simulink library "ILCUpdate"  (R2018a)
settings: Solver=VariableStepAuto  StartTime=0.0  StopTime=10.0  RelTol=1e-3
undefined symbols (not defined in the file or in its folder): ctrl
libraries: normalizeBasisParameters x2, updateLaw_cd x1, initializeResponseSurface_cd x1, manageILCTriggers_ul x1, updateResponseSurface_ul x1, normalizePerformanceIndex x1, rescaleBasisParameters x1
settings Model: Creator=mitch  LastModifiedBy=mitch

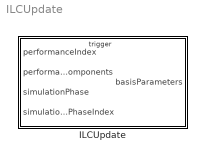
== system ILCUpdate ==
  ILCUpdate : Subsystem

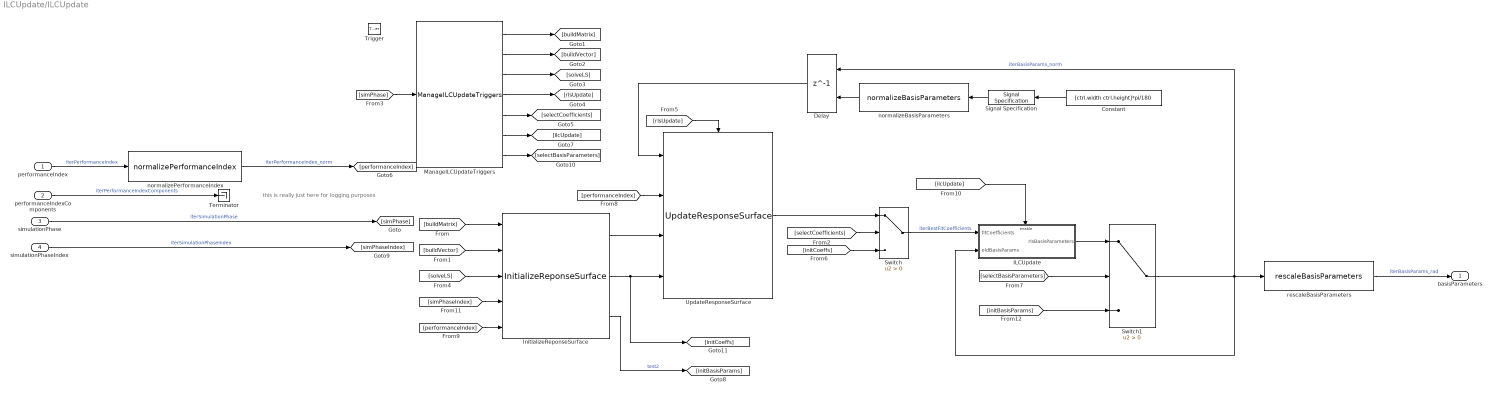
== system ILCUpdate/ILCUpdate ==
  note: this is really just here for logging purposes
  performanceIndex : Inport
  performanceIndexComponents : Inport  Port=2
  simulationPhase : Inport  Port=3  OutDataTypeStr=Enum: simulationPhase_enum
  simulationPhaseIndex : Inport  Port=4
  Trigger : TriggerPort  VariantControl=Variant  InitialTriggerSignalState=positive  PortDimensions=1
  Constant : Constant  Value=[ctrl.width ctrl.height]*pi/180
  Delay : Delay  DelayLength=1  InitialConditionSource=Input port
      settings: InputPortMap=u0,p4
  ILCUpdate : Subsystem
  InitializeReponseSurface : initializeResponseSurface_cd/InitializeReponseSurface
  ManageILCUpdateTriggers : manageILCTriggers_ul/ManageILCUpdateTriggers
  Signal Specification : SignalSpecification  Dimensions=[1 2]
  Switch : Switch  Criteria=u2 > Threshold
  Switch1 : Switch  Criteria=u2 > Threshold
  Terminator : Terminator
  UpdateResponseSurface : updateResponseSurface_ul/UpdateResponseSurface
  normalizeBasisParameters : normalizeBasisParameters/normalizeBasisParameters
  normalizePerformanceIndex : normalizePerformanceIndex/normalizePerformanceIndex
  rescaleBasisParameters : rescaleBasisParameters/rescaleBasisParameters
  basisParameters : Outport  InitialOutput=[ctrl.width ctrl.height]*pi/180
  wires:
  [initBasisParams] -> Switch1/3
  [selectBasisParameters] -> Switch1/2
  ILCUpdate/1(rlsBasisParameters) -> Switch1/1
  [ilcUpdate] -> ILCUpdate/Enable
  [initCoeffs] -> Switch/3
  UpdateResponseSurface/1 -> Switch/1
  [selectCoefficients] -> Switch/2
  [solveLS] -> InitializeReponseSurface/3
  [buildVector] -> InitializeReponseSurface/2
  [buildMatrix] -> InitializeReponseSurface/1
  ManageILCUpdateTriggers/7 -> [selectBasisParameters]
  ManageILCUpdateTriggers/6 -> [ilcUpdate]
  ManageILCUpdateTriggers/5 -> [selectCoefficients]
  ManageILCUpdateTriggers/4 -> [rlsUpdate]
  ManageILCUpdateTriggers/3 -> [solveLS]
  ManageILCUpdateTriggers/2 -> [buildVector]
  [performanceIndex] -> UpdateResponseSurface/2
  InitializeReponseSurface/3 -> [initBasisParams]  "test2"
  [performanceIndex] -> InitializeReponseSurface/5
  performanceIndex/1 -> normalizePerformanceIndex/1  "iterPerformanceIndex"
  InitializeReponseSurface/2 -> UpdateResponseSurface/4, [initCoeffs]
  InitializeReponseSurface/1 -> UpdateResponseSurface/3
  simulationPhase/1 -> [simPhase]  "iterSimulationPhase"
  [simPhase] -> ManageILCUpdateTriggers/1
  ManageILCUpdateTriggers/1 -> [buildMatrix]
  simulationPhaseIndex/1 -> [simPhaseIndex]  "iterSimulationPhaseIndex"
  [simPhaseIndex] -> InitializeReponseSurface/4
  Switch1/1 -> ILCUpdate/2(oldBasisParams), Delay/1, rescaleBasisParameters/1  "iterBasisParams_norm"
  Switch/1 -> ILCUpdate/1(fitCoefficients)  "iterBestFitCoefficients"
  [rlsUpdate] -> UpdateResponseSurface/Enable
  normalizePerformanceIndex/1 -> [performanceIndex]  "iterPerformanceIndex_norm"
  Delay/1 -> UpdateResponseSurface/1
  Constant/1 -> Signal Specification/1
  rescaleBasisParameters/1 -> basisParameters/1  "iterBasisParams_rad"
  Signal Specification/1 -> normalizeBasisParameters/1
  normalizeBasisParameters/1 -> Delay/2
  performanceIndexComponents/1 -> Terminator/1  "iterPerformanceIndexComponents"

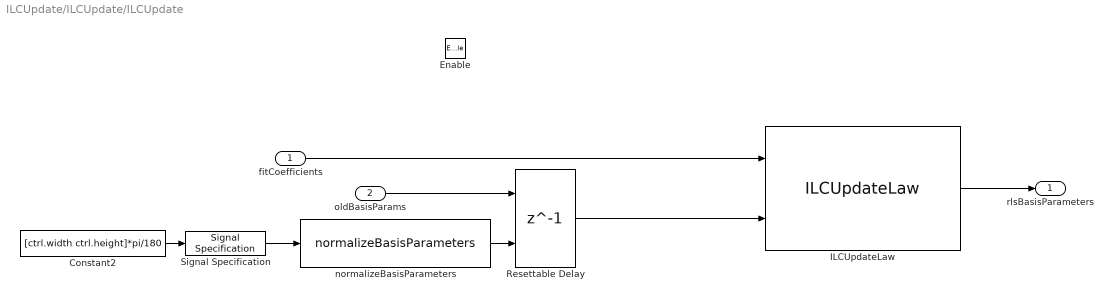
== system ILCUpdate/ILCUpdate/ILCUpdate ==
  fitCoefficients : Inport
  oldBasisParams : Inport  Port=2
  Enable : EnablePort
  Constant2 : Constant  Value=[ctrl.width ctrl.height]*pi/180
  ILCUpdateLaw : updateLaw_cd/ILCUpdateLaw
  Resettable Delay : Delay  DelayLength=1  InitialConditionSource=Input port
      settings: InputPortMap=u0,p4
  Signal Specification : SignalSpecification  Dimensions=[1 2]
  normalizeBasisParameters : normalizeBasisParameters/normalizeBasisParameters
  rlsBasisParameters : Outport  PortDimensions=[1 2]  SourceOfInitialOutputValue=Input signal  InitialOutput=[ctrl.width ctrl.height]*pi/180
  wires:
  ILCUpdateLaw/1 -> rlsBasisParameters/1
  fitCoefficients/1 -> ILCUpdateLaw/1
  oldBasisParams/1 -> Resettable Delay/1
  Constant2/1 -> Signal Specification/1
  Resettable Delay/1 -> ILCUpdateLaw/2
  normalizeBasisParameters/1 -> Resettable Delay/2
  Signal Specification/1 -> normalizeBasisParameters/1
